simulink model "RocketFlight_6DOF"  (R2014a)
settings: Solver=ode3  StartTime=0.0  StopTime=25  FixedStep=0.01  MinStep=0.01  RelTol=1e-3
undefined symbols (not defined in the file or in its folder): area_rocket_planform, distance_tip_to_COP, dry_rocket_cog, ground_launch_altitude, ground_pressure_ambient, ground_temperature_ambient, launch_angle, moment_inertia_rocket, wet_motor_mass
libraries: rocket_angular_flight_library x4, rocket_isa_model_library x2, rocket_drag_library x2, aerolib6dof2 x1, rocket_dynamic_data_library x1, rocket_vertical_flight_library x1
settings Model: Creator=scorpii  LastModifiedBy=scorpii
settings SolverCC: InitialStep=0.01
settings DataIOCC: LimitDataPoints=off
settings OptimizationCC: SimCompilerOptimization=off
settings DebuggingCC: ArtificialAlgebraicLoopMsg=error  MergeDetectMultiDrivingBlocksExec=error  FrameProcessingCompatibilityMsg=error
settings RTWCC: RTWCompilerOptimization=off

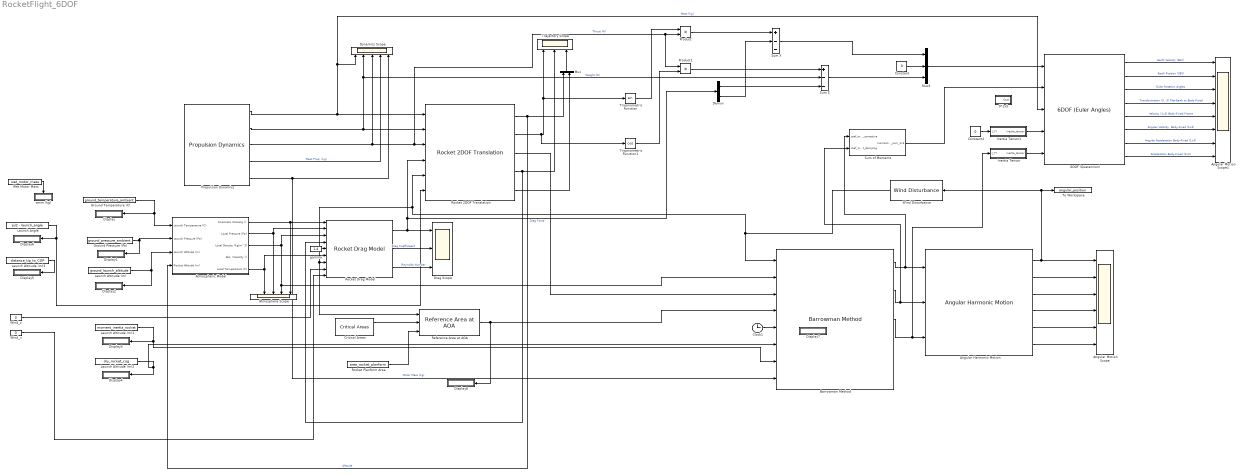
== system RocketFlight_6DOF ==
  " Launch Angle" : Constant  Value=pi/2 - launch_angle
  0*1x3 : Subsystem
  6DOF (Quaternion) : aerolib6dof2/6DOF (Euler Angles)  units=Metric (MKS)  mtype=Custom Variable  rep=Quaternion  xme_0=[0 0 0]  Vm_0=[0 0 0]  eul_0=[0 0.15708 0]  pm_0=[0 0 0]  mass_0=1.0  mass_e=0.5  mass_f=2.0  inertia=eye(3)  inertia_e=eye(3)  inertia_f=2*eye(3)  k_quat=1.0  vre_flag=off
  Angular Harmonic Motion : rocket_angular_flight_library/Shawn  Angular Flight Model/Shawn Angular Model/Angular Harmonic Motion
  Angular Motion Scope : Scope  NumInputPorts=6
      settings: TimeRange=10  YMin=-0.003~-0.0075~-0.04~0.067832~6.4~1.07  YMax=0.0025~0.0125~0.06~0.0678327~7.7~1.125  SaveName=ScopeData5
  Angular Motion Scope1 : Scope  NumInputPorts=8
      settings: TimeRange=10  YMin=-0.003~-0.0075~-0.04~0.067832~6.4~1.07~-5~-5  YMax=0.0025~0.0125~0.06~0.0678327~7.7~1.125~5~5  SaveName=ScopeData6
  Atmosphere Scope : Scope  NumInputPorts=5
      settings: YMin=-1~28.5~96258.8~11.1784~-1.12485e-07  YMax=1~31.5~106391~12.355~-1.01773e-07  SaveName=ScopeData4
  Atmospheric Model : Subsystem
  Barrowman Method : rocket_angular_flight_library/Shawn  Angular Flight Model/Shawn Angular Model/Barrowman Method
  Clock1 : Clock
  Constant : Constant  Value=0
  Constant2 : Constant  Value=0
  Critical Areas : rocket_drag_library/Critical Areas
  Demux : Demux  Outputs=2
  Display{,1..8} (9 alike) : Display
  Drag Scope : Scope  NumInputPorts=3
      settings: YMin=30~0.45~1.75e+07  YMax=240~0.725~5e+07  SaveName=ScopeData3
  Dynamics Scope : Scope  NumInputPorts=5
      settings: YMin=126.243~1238.44~774.486~-5~-5  YMax=139.531~1368.8~856.01~5~5
  Ground Pressure (Pa) : Constant  Value=ground_pressure_ambient
  Ground Temperature (C) : Constant  Value=ground_temperature_ambient
  Inertia Tensor : Subsystem
  Inertia Tensor1 : Subsystem
  Launch Altitude (m) : Constant  Value=ground_launch_altitude
  Launch Altitude (m)1 : Constant  Value=moment_inertia_rocket
  Launch Altitude (m)2 : Constant  Value=dry_rocket_cog
  Launch Altitude (m)3 : Constant  Value=distance_tip_to_COP
  Mux : Mux  Inputs=2
  Mux3 : Mux  Inputs=3
  Product : Product
  Product1 : Product
  Propulsion Dynamics : rocket_dynamic_data_library/Propulsion Dynamics
  Reference Area at AOA : rocket_angular_flight_library/Reference Area at AOA
  Rocket 2DOF Translation : rocket_vertical_flight_library/Rocket 2DOF Translation
  Rocket Drag Model : rocket_drag_library/Rocket Drag Model
  Rocket Planform Area : Constant  Value=area_rocket_planform
  Sum X : Sum  Inputs=+--
  Sum Z : Sum  Inputs=+--
  Sum of Moments : Subsystem
  To Workspace : ToWorkspace  VariableName=angular_position  SampleTime=-1
  Trajectory Scope : Scope  NumInputPorts=3
      settings: YMin=0.04~25~-1  YMax=0.145~525~1  SaveName=ScopeData7
  Trigonometric Function : Trigonometry
  Trigonometric Function1 : Trigonometry  Operator=cos
  Wet Motor Mass : Constant  Value=wet_motor_mass
  Wind Disturbance : rocket_angular_flight_library/Wind Disturbance
  Wind_x : Constant  Value=0
  Wind_z : Constant  Value=0
  gamma : Constant  Value=1.4
  wmm (kg) : Display
  wires:
  Angular Harmonic Motion/2 -> Angular Motion Scope/2
  Angular Harmonic Motion/3 -> Angular Motion Scope/3
  Angular Harmonic Motion/4 -> Angular Motion Scope/4
  Angular Harmonic Motion/5 -> Angular Motion Scope/5
  Angular Harmonic Motion/6 -> Angular Motion Scope/6
  Barrowman Method/1 -> Sum of Moments/1(coef_moment_corrective), Angular Harmonic Motion/1
  Barrowman Method/2 -> Sum of Moments/2(coef_moment_damping), Angular Harmonic Motion/2
  Angular Harmonic Motion/1 -> To Workspace/1, Wind Disturbance/1, Angular Motion Scope/1
  Sum Z/1 -> Mux3/3
  6DOF (Quaternion)/1 -> Angular Motion Scope1/1  "Earth Velocity (3EV)"
  6DOF (Quaternion)/8 -> Angular Motion Scope1/8  "Acceleration Body-Fixed (1x3)"
  6DOF (Quaternion)/6 -> Angular Motion Scope1/6  "Angular Velocity  Body-Fixed (1x3)"
  6DOF (Quaternion)/7 -> Angular Motion Scope1/7  "Angular Acceleration Body-Fixed (1x3)"
  6DOF (Quaternion)/2 -> Angular Motion Scope1/2  "Earth Position (3EV)"
  6DOF (Quaternion)/3 -> Angular Motion Scope1/3  "Euler Rotation Angles"
  6DOF (Quaternion)/4 -> Angular Motion Scope1/4  "Transformation (3x3) Flat-Earth to Body-Fixed"
  6DOF (Quaternion)/5 -> Angular Motion Scope1/5  "Velocity (1x3) Body-Fixed Frame"
  Sum of Moments/1(moments_sum_1x3) -> 6DOF (Quaternion)/2
  Barrowman Method/3 -> Inertia Tensor/1(I_YY), Angular Harmonic Motion/3
  Mux3/1 -> 6DOF (Quaternion)/1
  Inertia Tensor/1(inertia_tensor) -> 6DOF (Quaternion)/5
  Constant2/1 -> Inertia Tensor1/1(I_YY)
  Inertia Tensor1/1(inertia_tensor) -> 6DOF (Quaternion)/4
  Atmospheric Model/3(Local Density (kg/m^3)) -> Rocket Drag Model/3, Barrowman Method/2, Atmosphere Scope/4
  Atmospheric Model/2(Local Pressure (Pa)) -> Rocket Drag Model/2, Atmosphere Scope/3
  Atmospheric Model/1(Kinematic Viscosity ()) -> Rocket Drag Model/1, Atmosphere Scope/5
  Atmospheric Model/5(Local Temperature (K)) -> Rocket Drag Model/6, Atmosphere Scope/2
  Propulsion Dynamics/2 -> Dynamics Scope/2, Sum Z/2, Rocket 2DOF Translation/2  "Weight (N)"
  Propulsion Dynamics/3 -> Dynamics Scope/3, Product1/1, Product/2, Rocket 2DOF Translation/3  "Thrust (N)"
  gamma/1 -> Rocket Drag Model/5
  Ground Temperature (C)/1 -> Display/1, Atmospheric Model/1(Launch Temperature (C))
  Ground Pressure (Pa)/1 -> Display1/1, Atmospheric Model/2(Launch Pressure (Pa))
  Launch Altitude (m)/1 -> Atmospheric Model/3(Launch Altitude (m)), Display2/1
  Propulsion Dynamics/4 -> Dynamics Scope/4  "Mass Prop. (kg)"
  Launch Altitude (m)1/1 -> Barrowman Method/7, Display3/1
  Wind Disturbance/1 -> Barrowman Method/1, Reference Area at AOA/1, Rocket Drag Model/7, Rocket 2DOF Translation/5
  Launch Altitude (m)2/1 -> Barrowman Method/6, Display4/1
  Launch Altitude (m)3/1 -> Display5/1
  Rocket Planform Area/1 -> Reference Area at AOA/3
  Critical Areas/1 -> Reference Area at AOA/2
  " Launch Angle"/1 -> Display6/1, Rocket 2DOF Translation/6
  Wet Motor Mass/1 -> wmm (kg)/1
  Reference Area at AOA/1 -> Barrowman Method/4, Display8/1
  Propulsion Dynamics/5 -> Dynamics Scope/5, Barrowman Method/8  "Motor Mass (kg)"
  Propulsion Dynamics/1 -> Rocket 2DOF Translation/1, 6DOF (Quaternion)/3, Dynamics Scope/1  "Mass (kg)"
  Rocket Drag Model/1 -> Rocket 2DOF Translation/4, Demux/1, Drag Scope/1  "Drag Force"
  Rocket Drag Model/2 -> Drag Scope/2  "Drag Coefficieent"
  Rocket Drag Model/3 -> Drag Scope/3  "Reynolds Number"
  Wind_x/1 -> Rocket Drag Model/9
  Wind_z/1 -> Rocket Drag Model/8
  Rocket 2DOF Translation/2 -> Trigonometric Function1/1, Trigonometric Function/1, Trajectory Scope/1
  Rocket 2DOF Translation/5 -> Mux/2
  Rocket 2DOF Translation/4 -> Trajectory Scope/2, Rocket Drag Model/4
  Rocket 2DOF Translation/3 -> Barrowman Method/3
  Clock1/1 -> Barrowman Method/5
  Rocket 2DOF Translation/1 -> Atmospheric Model/4(Rocket Altitude (m)), Mux/1  "Altitude"
  Mux/1 -> Trajectory Scope/3
  Demux/1 -> Sum Z/3
  Demux/2 -> Sum X/2
  Trigonometric Function/1 -> Product/1
  Product/1 -> Sum X/1
  Trigonometric Function1/1 -> Product1/2
  Product1/1 -> Sum Z/1
  Constant/1 -> Mux3/2
  Sum X/1 -> Mux3/1

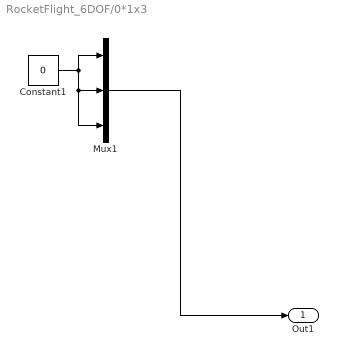
== system RocketFlight_6DOF/0*1x3 ==
  Constant1 : Constant  Value=0
  Mux1 : Mux  Inputs=3
  Out1 : Outport
  wires:
  Mux1/1 -> Out1/1
  Constant1/1 -> Mux1/1, Mux1/3, Mux1/2

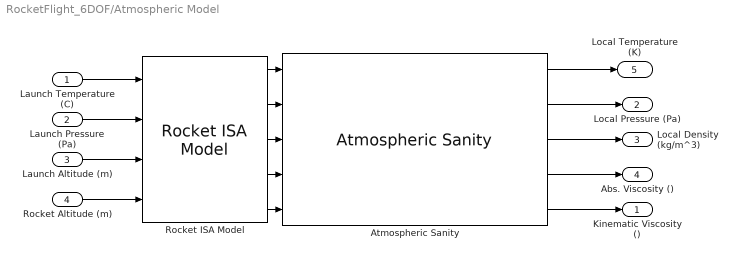
== system RocketFlight_6DOF/Atmospheric Model ==
  Launch Temperature (C) : Inport
  Launch Pressure (Pa) : Inport  Port=2
  Launch Altitude (m) : Inport  Port=3
  Rocket Altitude (m) : Inport  Port=4
  Atmospheric Sanity : rocket_isa_model_library/Atmospheric Sanity
  Rocket ISA Model : rocket_isa_model_library/Rocket ISA Model
  Kinematic Viscosity () : Outport
  Local Pressure (Pa) : Outport  Port=2
  Local Density (kg/m^3) : Outport  Port=3
  Abs. Viscosity () : Outport  Port=4
  Local Temperature (K) : Outport  Port=5
  wires:
  Rocket ISA Model/5 -> Atmospheric Sanity/5
  Rocket ISA Model/2 -> Atmospheric Sanity/2
  Rocket ISA Model/3 -> Atmospheric Sanity/3
  Atmospheric Sanity/2 -> Local Pressure (Pa)/1
  Rocket ISA Model/4 -> Atmospheric Sanity/4
  Atmospheric Sanity/5 -> Kinematic Viscosity ()/1
  Atmospheric Sanity/1 -> Local Temperature (K)/1
  Atmospheric Sanity/3 -> Local Density (kg/m^3)/1
  Rocket ISA Model/1 -> Atmospheric Sanity/1
  Launch Temperature (C)/1 -> Rocket ISA Model/1
  Atmospheric Sanity/4 -> Abs. Viscosity ()/1
  Launch Pressure (Pa)/1 -> Rocket ISA Model/2
  Launch Altitude (m)/1 -> Rocket ISA Model/3
  Rocket Altitude (m)/1 -> Rocket ISA Model/4

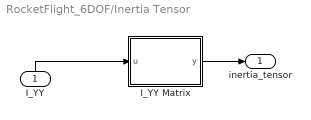
== system RocketFlight_6DOF/Inertia Tensor ==
  I_YY : Inport
  I_YY Matrix : MATLAB Function  TreatAsAtomicUnit=on
  inertia_tensor : Outport
  wires:
  I_YY Matrix/1(y) -> inertia_tensor/1
  I_YY/1 -> I_YY Matrix/1(u)

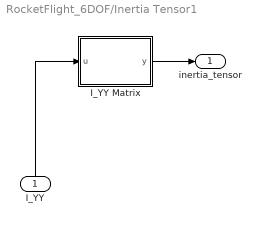
== system RocketFlight_6DOF/Inertia Tensor1 ==
  I_YY : Inport
  I_YY Matrix : MATLAB Function  TreatAsAtomicUnit=on
  inertia_tensor : Outport
  wires:
  I_YY Matrix/1(y) -> inertia_tensor/1
  I_YY/1 -> I_YY Matrix/1(u)

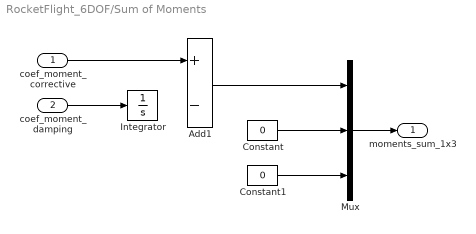
== system RocketFlight_6DOF/Sum of Moments ==
  coef_moment_corrective : Inport
  coef_moment_damping : Inport  Port=2
  Add1 : Sum  Inputs=+-
  Constant : Constant  Value=0
  Constant1 : Constant  Value=0
  Integrator : Integrator
  Mux : Mux  Inputs=3
  moments_sum_1x3 : Outport
  wires:
  coef_moment_corrective/1 -> Add1/1
  Mux/1 -> moments_sum_1x3/1
  coef_moment_damping/1 -> Integrator/1
  Constant1/1 -> Mux/3
  Constant/1 -> Mux/2
  Add1/1 -> Mux/1

== matlab function RocketFlight_6DOF/Inertia Tensor1/I_YY Matrix ==
  data: u input; y output
function y = fcn(u)
y = [ u 0 0; 0 0 0; 0 0 0 ];

== matlab function RocketFlight_6DOF/Inertia Tensor/I_YY Matrix ==
  data: u input; y output
function y = fcn(u)
y = [ 1 0 0; 0 u 0; 0 0 1 ];
